simulink model "OPENXWD"  (R2022b)
settings: Solver=VariableStepAuto  StartTime=0.0  StopTime=inf  RelTol=1e-3  EnableMultiTasking=on
PreLoadFcn:
  | run('Parameters\FSE_Parameters.m')
values from neighbouring files (symbols this model uses):
  batt_curr = 1    [srcipt.m]
  batt_voltage = 587    [srcipt.m]
  drive_ratio = 14.25    [srcipt.m]
  g = 9.81    [srcipt.m]
  h = 0.25    [srcipt.m]
  Ku = 1/500*-1    (= -0.002)    [srcipt.m]
  L = 1.53    [srcipt.m]
  lf = L-lr    (= 0.765)    [srcipt.m]
  lr = 0.765    [srcipt.m]
  ls = 1.242    [srcipt.m]
  m = 226    [srcipt.m]
  max_moment = 9.8    [srcipt.m]
  Mz_I = 70    [srcipt.m]
  Mz_p = 700    [srcipt.m]
  P_max = 80000    [srcipt.m]
  rw = 0.217    [srcipt.m]
libraries: CarMaker4SL x44, simulink x1
(part 2 of 3)

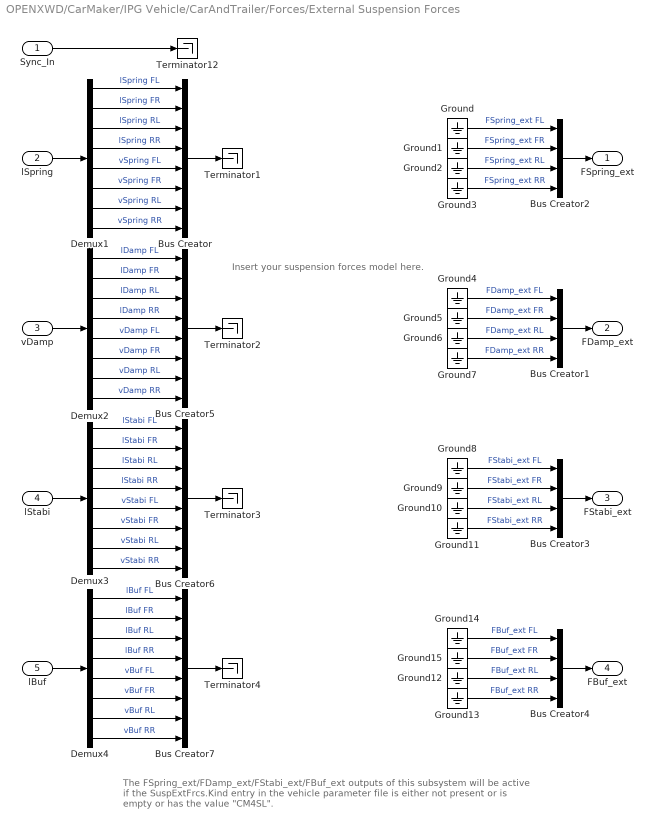
== system OPENXWD/CarMaker/IPG Vehicle/CarAndTrailer/Forces/External Suspension Forces ==
  note: The FSpring_ext/FDamp_ext/FStabi_ext/FBuf_ext outputs of this subsystem will be
      | active if the SuspExtFrcs.Kind entry in the vehicle parameter file
      | is either not present or is empty or has the value "CM4SL".
  note: Insert your suspension forces model here.
  Sync_In : Inport
  lSpring : Inport  Port=2
  vDamp : Inport  Port=3
  lStabi : Inport  Port=4
  lBuf : Inport  Port=5
  Bus Creator{,5..7} (4 alike) : BusCreator  Inputs=8
  Bus Creator{1..4} (4 alike) : BusCreator  Inputs=4
  Demux{1..4} (4 alike) : Demux  Outputs=8
      settings: DisplayOption=none
  Ground{,1..15} (16 alike) : Ground
  Terminator{1..4,12} (5 alike) : Terminator
  FSpring_ext : Outport
  FDamp_ext : Outport  Port=2
  FStabi_ext : Outport  Port=3
  FBuf_ext : Outport  Port=4
  wires:
  Bus Creator7/1 -> Terminator4/1
  Bus Creator6/1 -> Terminator3/1
  Bus Creator5/1 -> Terminator2/1
  Bus Creator/1 -> Terminator1/1
  Demux4/8 -> Bus Creator7/8  "vBuf RR"
  Demux4/7 -> Bus Creator7/7  "vBuf RL"
  Demux4/6 -> Bus Creator7/6  "vBuf FR"
  Demux4/5 -> Bus Creator7/5  "vBuf FL"
  Demux3/8 -> Bus Creator6/8  "vStabi RR"
  Demux3/7 -> Bus Creator6/7  "vStabi RL"
  Demux3/6 -> Bus Creator6/6  "vStabi FR"
  Demux3/5 -> Bus Creator6/5  "vStabi FL"
  Demux2/8 -> Bus Creator5/8  "vDamp RR"
  Demux2/7 -> Bus Creator5/7  "vDamp RL"
  Demux2/6 -> Bus Creator5/6  "vDamp FR"
  Demux2/5 -> Bus Creator5/5  "vDamp FL"
  Demux1/8 -> Bus Creator/8  "vSpring RR"
  Demux1/7 -> Bus Creator/7  "vSpring RL"
  Demux1/6 -> Bus Creator/6  "vSpring FR"
  Demux1/5 -> Bus Creator/5  "vSpring FL"
  Demux2/4 -> Bus Creator5/4  "lDamp RR"
  Demux2/3 -> Bus Creator5/3  "lDamp RL"
  Demux2/2 -> Bus Creator5/2  "lDamp FR"
  Demux2/1 -> Bus Creator5/1  "lDamp FL"
  Demux1/4 -> Bus Creator/4  "lSpring RR"
  Demux1/3 -> Bus Creator/3  "lSpring RL"
  Demux1/2 -> Bus Creator/2  "lSpring FR"
  Demux1/1 -> Bus Creator/1  "lSpring FL"
  Demux3/4 -> Bus Creator6/4  "lStabi RR"
  Demux3/3 -> Bus Creator6/3  "lStabi RL"
  Demux3/2 -> Bus Creator6/2  "lStabi FR"
  Demux3/1 -> Bus Creator6/1  "lStabi FL"
  lStabi/1 -> Demux3/1
  vDamp/1 -> Demux2/1
  lSpring/1 -> Demux1/1
  Demux4/4 -> Bus Creator7/4  "lBuf RR"
  Demux4/3 -> Bus Creator7/3  "lBuf RL"
  Demux4/2 -> Bus Creator7/2  "lBuf FR"
  Demux4/1 -> Bus Creator7/1  "lBuf FL"
  lBuf/1 -> Demux4/1
  Ground14/1 -> Bus Creator4/1  "FBuf_ext FL"
  Ground15/1 -> Bus Creator4/2  "FBuf_ext FR"
  Ground12/1 -> Bus Creator4/3  "FBuf_ext RL"
  Ground13/1 -> Bus Creator4/4  "FBuf_ext RR"
  Bus Creator4/1 -> FBuf_ext/1
  Sync_In/1 -> Terminator12/1
  Bus Creator2/1 -> FSpring_ext/1
  Ground/1 -> Bus Creator2/1  "FSpring_ext FL"
  Ground1/1 -> Bus Creator2/2  "FSpring_ext FR"
  Ground2/1 -> Bus Creator2/3  "FSpring_ext RL"
  Ground3/1 -> Bus Creator2/4  "FSpring_ext RR"
  Ground4/1 -> Bus Creator1/1  "FDamp_ext FL"
  Ground5/1 -> Bus Creator1/2  "FDamp_ext FR"
  Ground6/1 -> Bus Creator1/3  "FDamp_ext RL"
  Ground7/1 -> Bus Creator1/4  "FDamp_ext RR"
  Bus Creator1/1 -> FDamp_ext/1
  Ground8/1 -> Bus Creator3/1  "FStabi_ext FL"
  Ground9/1 -> Bus Creator3/2  "FStabi_ext FR"
  Ground10/1 -> Bus Creator3/3  "FStabi_ext RL"
  Ground11/1 -> Bus Creator3/4  "FStabi_ext RR"
  Bus Creator3/1 -> FStabi_ext/1

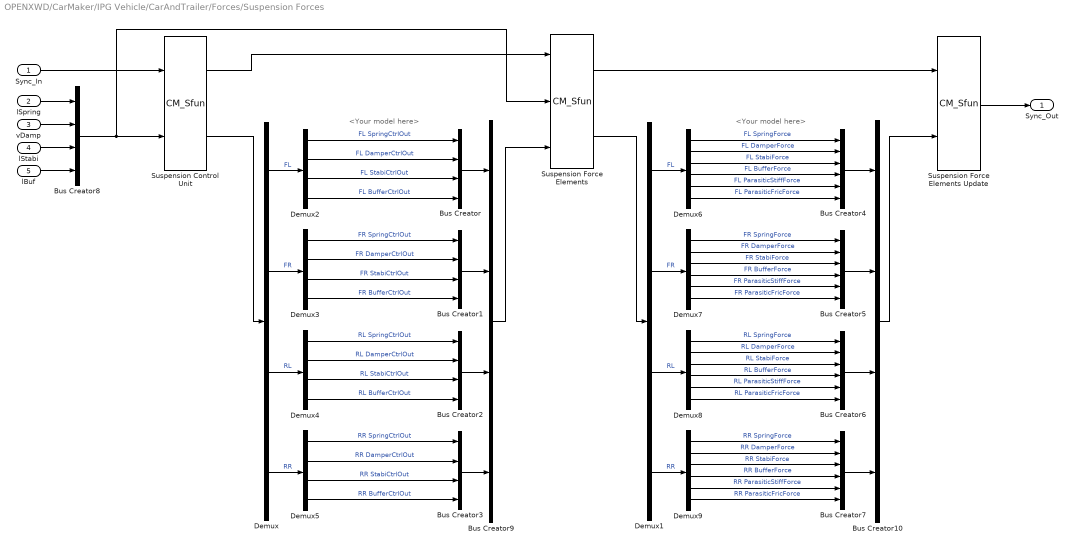
== system OPENXWD/CarMaker/IPG Vehicle/CarAndTrailer/Forces/Suspension Forces ==
  note: <Your model here>
  note: <Your model here>
  Sync_In : Inport
  lSpring : Inport  Port=2
  vDamp : Inport  Port=3
  lStabi : Inport  Port=4
  lBuf : Inport  Port=5
  Bus Creator{,1..3,8..10} (7 alike) : BusCreator  Inputs=4
  Bus Creator{4..7} (4 alike) : BusCreator  Inputs=6
  Demux{,1..5} (6 alike) : Demux
  Demux{6..9} (4 alike) : Demux  Outputs=6
  Suspension Control Unit : S-Function  FunctionName=CM_Sfun  Parameters='ForcesSuspControl'  SFunctionDeploymentMode=off  EnableBusSupport=off
  Suspension Force Elements : S-Function  FunctionName=CM_Sfun  Parameters='ForcesSusp'  SFunctionDeploymentMode=off  EnableBusSupport=off
  Suspension Force Elements Update : S-Function  FunctionName=CM_Sfun  Parameters='ForcesSuspUpd'  SFunctionDeploymentMode=off  EnableBusSupport=off
  Sync_Out : Outport
  wires:
  vDamp/1 -> Bus Creator8/2
  lStabi/1 -> Bus Creator8/3
  lBuf/1 -> Bus Creator8/4
  lSpring/1 -> Bus Creator8/1
  Bus Creator8/1 -> Suspension Control Unit/2, Suspension Force Elements/2
  Sync_In/1 -> Suspension Control Unit/1
  Suspension Control Unit/1 -> Suspension Force Elements/1
  Suspension Force Elements/1 -> Suspension Force Elements Update/1
  Suspension Force Elements Update/1 -> Sync_Out/1
  Bus Creator4/1 -> Bus Creator10/1
  Bus Creator5/1 -> Bus Creator10/2
  Bus Creator6/1 -> Bus Creator10/3
  Bus Creator7/1 -> Bus Creator10/4
  Demux6/1 -> Bus Creator4/1  "FL SpringForce"
  Demux9/1 -> Bus Creator7/1  "RR SpringForce"
  Demux9/2 -> Bus Creator7/2  "RR DamperForce"
  Demux9/3 -> Bus Creator7/3  "RR StabiForce"
  Demux9/4 -> Bus Creator7/4  "RR BufferForce"
  Demux9/5 -> Bus Creator7/5  "RR ParasiticStiffForce"
  Demux9/6 -> Bus Creator7/6  "RR ParasiticFricForce"
  Demux8/1 -> Bus Creator6/1  "RL SpringForce"
  Demux8/2 -> Bus Creator6/2  "RL DamperForce"
  Demux8/4 -> Bus Creator6/4  "RL BufferForce"
  Demux8/5 -> Bus Creator6/5  "RL ParasiticStiffForce"
  Demux8/6 -> Bus Creator6/6  "RL ParasiticFricForce"
  Demux8/3 -> Bus Creator6/3  "RL StabiForce"
  Demux7/1 -> Bus Creator5/1  "FR SpringForce"
  Demux7/2 -> Bus Creator5/2  "FR DamperForce"
  Demux7/3 -> Bus Creator5/3  "FR StabiForce"
  Demux7/4 -> Bus Creator5/4  "FR BufferForce"
  Demux7/5 -> Bus Creator5/5  "FR ParasiticStiffForce"
  Demux7/6 -> Bus Creator5/6  "FR ParasiticFricForce"
  Demux6/2 -> Bus Creator4/2  "FL DamperForce"
  Demux6/3 -> Bus Creator4/3  "FL StabiForce"
  Demux6/4 -> Bus Creator4/4  "FL BufferForce"
  Demux6/5 -> Bus Creator4/5  "FL ParasiticStiffForce"
  Demux6/6 -> Bus Creator4/6  "FL ParasiticFricForce"
  Bus Creator10/1 -> Suspension Force Elements Update/2
  Demux/1 -> Demux2/1  "FL"
  Bus Creator1/1 -> Bus Creator9/2
  Demux/2 -> Demux3/1  "FR"
  Bus Creator2/1 -> Bus Creator9/3
  Demux/3 -> Demux4/1  "RL"
  Bus Creator3/1 -> Bus Creator9/4
  Demux2/1 -> Bus Creator/1  "FL SpringCtrlOut"
  Demux/4 -> Demux5/1  "RR"
  Demux5/1 -> Bus Creator3/1  "RR SpringCtrlOut"
  Demux5/2 -> Bus Creator3/2  "RR DamperCtrlOut"
  Demux5/3 -> Bus Creator3/3  "RR StabiCtrlOut"
  Demux5/4 -> Bus Creator3/4  "RR BufferCtrlOut"
  Demux4/1 -> Bus Creator2/1  "RL SpringCtrlOut"
  Demux4/2 -> Bus Creator2/2  "RL DamperCtrlOut"
  Demux4/4 -> Bus Creator2/4  "RL BufferCtrlOut"
  Demux4/3 -> Bus Creator2/3  "RL StabiCtrlOut"
  Demux3/1 -> Bus Creator1/1  "FR SpringCtrlOut"
  Demux3/2 -> Bus Creator1/2  "FR DamperCtrlOut"
  Demux3/3 -> Bus Creator1/3  "FR StabiCtrlOut"
  Demux3/4 -> Bus Creator1/4  "FR BufferCtrlOut"
  Demux2/2 -> Bus Creator/2  "FL DamperCtrlOut"
  Demux2/3 -> Bus Creator/3  "FL StabiCtrlOut"
  Demux2/4 -> Bus Creator/4  "FL BufferCtrlOut"
  Suspension Control Unit/2 -> Demux/1
  Bus Creator9/1 -> Suspension Force Elements/3
  Bus Creator/1 -> Bus Creator9/1
  Suspension Force Elements/2 -> Demux1/1
  Demux1/1 -> Demux6/1  "FL"
  Demux1/2 -> Demux7/1  "FR"
  Demux1/3 -> Demux8/1  "RL"
  Demux1/4 -> Demux9/1  "RR"

== system OPENXWD/CarMaker/IPG Vehicle/CarAndTrailer/Forces/Tires ==
  note: The TireXX_Out signals will only be used if FileIdent is "CarMaker-Tire-CM4SL" in the tire parameter file!
      | An example parameter file can be found in Data/Tire/DT_CM4SL_UserTire.
  Sync_In : Inport
  TireFL_In : Inport  Port=2
  TireFR_In : Inport  Port=3
  TireRL_In : Inport  Port=4
  TireRR_In : Inport  Port=5
  Bus Creator{1..4} (4 alike) : BusCreator  Inputs=11
  Demux{1..3,8} (4 alike) : Demux  Outputs=7
      settings: DisplayOption=none
  TireFL : Subsystem
  TireFR : Subsystem
  TireRL : Subsystem
  TireRR : Subsystem
  TireFL_Out : Outport
  TireFR_Out : Outport  Port=2
  TireRL_Out : Outport  Port=3
  TireRR_Out : Outport  Port=4
  wires:
  Sync_In/1 -> TireRR/1(Sync_In), TireRL/1(Sync_In), TireFR/1(Sync_In), TireFL/1(Sync_In)
  Bus Creator4/1 -> TireRR_Out/1
  Bus Creator2/1 -> TireRL_Out/1
  Bus Creator1/1 -> TireFR_Out/1
  Demux3/5 -> TireRR/6(Rim_turnv)  "Tire_In Rim_turnv"
  Demux3/4 -> TireRR/5(Rim_rotv)  "Tire_In Rim_rotv"
  Demux3/1 -> TireRR/2(Load)  "Tire_In Load"
  Demux3/7 -> TireRR/8(muRoad)  "Tire_In mu"
  Demux3/6 -> TireRR/7(InclinAngle)  "Tire_In Camber"
  Demux3/2 -> TireRR/3(vxtrans)  "Tire_In vxtrans"
  Demux3/3 -> TireRR/4(vytrans)  "Tire_In vytrans"
  TireRR/11(AlignTrq) -> Bus Creator4/11  "Tire_Out AlignTrq"
  TireRR/10(RollResist) -> Bus Creator4/10  "Tire_Out RollResist"
  TireRR/9(OverturnTrq) -> Bus Creator4/9  "Tire_Out OverturnTrq"
  TireRR/8(LoadFrc) -> Bus Creator4/8  "Tire_Out LoadFrc"
  TireRR/7(SideFrc) -> Bus Creator4/7  "Tire_Out SideFrc"
  TireRR/6(LongFrc) -> Bus Creator4/6  "Tire_Out LongFrc"
  TireRR/5(vBelt) -> Bus Creator4/5  "Tire_Out vBelt"
  TireRR/4(rBelt_eff) -> Bus Creator4/4  "Tire_Out rBelt_eff"
  TireRR/3(TurnSlp) -> Bus Creator4/3  "Tire_Out TurnSlp"
  TireRR/1(Slp) -> Bus Creator4/1  "Tire_Out Slp"
  TireRR/2(Alpha) -> Bus Creator4/2  "Tire_Out Alpha"
  Demux2/5 -> TireRL/6(Rim_turnv)  "Tire_In Rim_turnv"
  Demux2/4 -> TireRL/5(Rim_rotv)  "Tire_In Rim_rotv"
  Demux2/1 -> TireRL/2(Load)  "Tire_In Load"
  Demux2/7 -> TireRL/8(muRoad)  "Tire_In mu"
  Demux2/6 -> TireRL/7(InclinAngle)  "Tire_In Camber"
  Demux2/2 -> TireRL/3(vxtrans)  "Tire_In vxtrans"
  Demux2/3 -> TireRL/4(vytrans)  "Tire_In vytrans"
  TireRL/11(AlignTrq) -> Bus Creator2/11  "Tire_Out AlignTrq"
  TireRL/10(RollResist) -> Bus Creator2/10  "Tire_Out RollResist"
  TireRL/9(OverturnTrq) -> Bus Creator2/9  "Tire_Out OverturnTrq"
  TireRL/8(LoadFrc) -> Bus Creator2/8  "Tire_Out LoadFrc"
  TireRL/7(SideFrc) -> Bus Creator2/7  "Tire_Out SideFrc"
  TireRL/6(LongFrc) -> Bus Creator2/6  "Tire_Out LongFrc"
  TireRL/5(vBelt) -> Bus Creator2/5  "Tire_Out vBelt"
  TireRL/4(rBelt_eff) -> Bus Creator2/4  "Tire_Out rBelt_eff"
  TireRL/3(TurnSlp) -> Bus Creator2/3  "Tire_Out TurnSlp"
  TireRL/1(Slp) -> Bus Creator2/1  "Tire_Out Slp"
  TireRL/2(Alpha) -> Bus Creator2/2  "Tire_Out Alpha"
  Demux1/5 -> TireFR/6(Rim_turnv)  "Tire_In Rim_turnv"
  Demux1/4 -> TireFR/5(Rim_rotv)  "Tire_In Rim_rotv"
  Demux1/1 -> TireFR/2(Load)  "Tire_In Load"
  Demux1/7 -> TireFR/8(muRoad)  "Tire_In mu"
  Demux1/6 -> TireFR/7(InclinAngle)  "Tire_In Camber"
  Demux1/2 -> TireFR/3(vxtrans)  "Tire_In vxtrans"
  Demux1/3 -> TireFR/4(vytrans)  "Tire_In vytrans"
  TireFR/11(AlignTrq) -> Bus Creator1/11  "Tire_Out AlignTrq"
  TireFR/10(RollResist) -> Bus Creator1/10  "Tire_Out RollResist"
  TireFR/9(OverturnTrq) -> Bus Creator1/9  "Tire_Out OverturnTrq"
  TireFR/8(LoadFrc) -> Bus Creator1/8  "Tire_Out LoadFrc"
  TireFR/7(SideFrc) -> Bus Creator1/7  "Tire_Out SideFrc"
  TireFR/6(LongFrc) -> Bus Creator1/6  "Tire_Out LongFrc"
  TireFR/5(vBelt) -> Bus Creator1/5  "Tire_Out vBelt"
  TireFR/4(rBelt_eff) -> Bus Creator1/4  "Tire_Out rBelt_eff"
  TireFR/3(TurnSlp) -> Bus Creator1/3  "Tire_Out TurnSlp"
  TireFR/1(Slp) -> Bus Creator1/1  "Tire_Out Slp"
  TireFR/2(Alpha) -> Bus Creator1/2  "Tire_Out Alpha"
  Demux8/5 -> TireFL/6(Rim_turnv)  "Tire_In Rim_turnv"
  Demux8/4 -> TireFL/5(Rim_rotv)  "Tire_In Rim_rotv"
  TireFL_In/1 -> Demux8/1
  Demux8/1 -> TireFL/2(Load)  "Tire_In Load"
  Demux8/7 -> TireFL/8(muRoad)  "Tire_In mu"
  Demux8/6 -> TireFL/7(InclinAngle)  "Tire_In Camber"
  Demux8/2 -> TireFL/3(vxtrans)  "Tire_In vxtrans"
  Demux8/3 -> TireFL/4(vytrans)  "Tire_In vytrans"
  TireFL/11(AlignTrq) -> Bus Creator3/11  "Tire_Out AlignTrq"
  TireFL/10(RollResist) -> Bus Creator3/10  "Tire_Out RollResist"
  TireFL/9(OverturnTrq) -> Bus Creator3/9  "Tire_Out OverturnTrq"
  TireFL/8(LoadFrc) -> Bus Creator3/8  "Tire_Out LoadFrc"
  TireFL/7(SideFrc) -> Bus Creator3/7  "Tire_Out SideFrc"
  TireFL/6(LongFrc) -> Bus Creator3/6  "Tire_Out LongFrc"
  TireFL/5(vBelt) -> Bus Creator3/5  "Tire_Out vBelt"
  TireFL/4(rBelt_eff) -> Bus Creator3/4  "Tire_Out rBelt_eff"
  TireFL/3(TurnSlp) -> Bus Creator3/3  "Tire_Out TurnSlp"
  TireFL/1(Slp) -> Bus Creator3/1  "Tire_Out Slp"
  TireFL/2(Alpha) -> Bus Creator3/2  "Tire_Out Alpha"
  Bus Creator3/1 -> TireFL_Out/1
  TireFR_In/1 -> Demux1/1
  TireRL_In/1 -> Demux2/1
  TireRR_In/1 -> Demux3/1

== system OPENXWD/CarMaker/IPG Vehicle/CarAndTrailer/Forces/Vehicle Forces ==
  Sync_In : Inport
  Bus Creator1 : BusCreator  Inputs=12
  Bus Creator8 : BusCreator  Inputs=16
  BusCreator1 : BusCreator  Inputs=4
  BusCreator2 : BusCreator  Inputs=9
  DRS_Example : Subsystem
  Demux : Demux  Outputs=16
      settings: DisplayOption=none
  Demux1 : Demux  Outputs=12
      settings: DisplayOption=none
  Demux2 : Demux  Outputs=13
      settings: DisplayOption=none
  Forces : S-Function  FunctionName=CM_Sfun  Parameters='Forces'  SFunctionDeploymentMode=off  EnableBusSupport=off
  Terminator : Terminator
  Sync_Out : Outport
  Car.Virtual : Outport  Port=2
  Car.Aero : Outport  Port=3
  Car.Load : Outport  Port=4
  wires:
  BusCreator1/1 -> Terminator/1  "Aero IF (in)"
  Demux2/13 -> BusCreator2/9  "car Aero Trq_1 z"
  Demux2/12 -> BusCreator2/8  "car Aero Trq_1 y"
  Demux2/11 -> BusCreator2/7  "car Aero Trq_1 x"
  Demux2/7 -> BusCreator2/3  "car Aero PoA_1 z"
  Demux2/6 -> BusCreator2/2  "car Aero PoA_1 y"
  Demux2/5 -> BusCreator2/1  "car Aero PoA_1 x"
  Demux2/4 -> BusCreator1/4  "car Aero tau_1"
  Demux2/3 -> BusCreator1/3  "car Aero ApproachVel_1 z"
  Demux2/2 -> BusCreator1/2  "car Aero ApproachVel_1 y"
  Demux2/1 -> BusCreator1/1  "car Aero ApproachVel_1 x"
  Demux/16 -> Bus Creator8/16  "Car Load_3 tz"
  Demux/15 -> Bus Creator8/15  "Car Load_3 ty"
  Demux/14 -> Bus Creator8/14  "Car Load_3 tx"
  Demux/13 -> Bus Creator8/13  "Car Load_3 mass"
  Demux1/12 -> Bus Creator1/12  "Car Virtual Trq_0 z"
  Demux1/11 -> Bus Creator1/11  "Car Virtual Trq_0 y"
  Demux1/10 -> Bus Creator1/10  "Car Virtual Trq_0 x"
  Demux1/9 -> Bus Creator1/9  "Car Virtual Trq_1 z"
  Demux1/8 -> Bus Creator1/8  "Car Virtual Trq_1 y"
  Demux1/7 -> Bus Creator1/7  "Car Virtual Trq_1 x"
  Demux1/6 -> Bus Creator1/6  "Car Virtual Frc_0 z"
  Demux1/5 -> Bus Creator1/5  "Car Virtual Frc_0 y"
  Demux1/4 -> Bus Creator1/4  "Car Virtual Frc_0 x"
  Sync_In/1 -> Forces/1
  Forces/1 -> Sync_Out/1
  BusCreator2/1 -> Car.Aero/1
  Demux1/1 -> Bus Creator1/1  "Car Virtual Frc_1 x"
  Demux1/2 -> Bus Creator1/2  "Car Virtual Frc_1 y"
  Demux1/3 -> Bus Creator1/3  "Car Virtual Frc_1 z"
  Forces/3 -> Demux2/1
  Forces/2 -> Demux1/1
  Bus Creator1/1 -> Car.Virtual/1
  Bus Creator8/1 -> Car.Load/1
  Demux/1 -> Bus Creator8/1  "Car Load_0 mass"
  Demux/2 -> Bus Creator8/2  "Car Load_0 tx"
  Demux/3 -> Bus Creator8/3  "Car Load_0 ty"
  Demux/4 -> Bus Creator8/4  "Car Load_0 tz"
  Demux/5 -> Bus Creator8/5  "Car Load_1 mass"
  Demux/6 -> Bus Creator8/6  "Car Load_1 tx"
  Demux/7 -> Bus Creator8/7  "Car Load_1 ty"
  Demux/8 -> Bus Creator8/8  "Car Load_1 tz"
  Demux/9 -> Bus Creator8/9  "Car Load_2 mass"
  Demux/10 -> Bus Creator8/10  "Car Load_2 tx"
  Demux/11 -> Bus Creator8/11  "Car Load_2 ty"
  Demux/12 -> Bus Creator8/12  "Car Load_2 tz"
  Forces/4 -> Demux/1
  DRS_Example/1(Car Aero Frc_1x) -> BusCreator2/4
  DRS_Example/2(Car Aero Frc_1y) -> BusCreator2/5
  DRS_Example/3(Car Aero Frc_1z) -> BusCreator2/6

== system OPENXWD/CarMaker/IPG Vehicle/CarAndTrailer/Trailer/CreateBus Car.Hitch.FrcTrq ==
  In1 : Inport
  Bus Creator7 : BusCreator  Inputs=6
  Demux7 : Demux  Outputs=6
      settings: DisplayOption=none
  Out1 : Outport
  wires:
  In1/1 -> Demux7/1
  Bus Creator7/1 -> Out1/1
  Demux7/6 -> Bus Creator7/6  "Car Hitch Trq2Car z"
  Demux7/5 -> Bus Creator7/5  "Car Hitch Trq2Car y"
  Demux7/4 -> Bus Creator7/4  "Car Hitch Trq2Car x"
  Demux7/3 -> Bus Creator7/3  "Car Hitch Frc2Car z"
  Demux7/2 -> Bus Creator7/2  "Car Hitch Frc2Car y"
  Demux7/1 -> Bus Creator7/1  "Car Hitch Frc2Car x"

== system OPENXWD/CarMaker/IPG Vehicle/CarAndTrailer/Trailer/CreateBus Vhcl.Motion ==
  In1 : Inport
  BusCreator : BusCreator  Inputs=15
  Demux : Demux  Outputs=15
      settings: DisplayOption=none
  Out1 : Outport
  wires:
  Demux/15 -> BusCreator/15  "Vhcl YawAcc"
  Demux/14 -> BusCreator/14  "Vhcl YawVel"
  Demux/13 -> BusCreator/13  "Vhcl Yaw"
  Demux/12 -> BusCreator/12  "Vhcl PitchAcc"
  Demux/11 -> BusCreator/11  "Vhcl PitchVel"
  Demux/10 -> BusCreator/10  "Vhcl Pitch"
  Demux/9 -> BusCreator/9  "Vhcl RollAcc"
  Demux/8 -> BusCreator/8  "Vhcl RollVel"
  Demux/7 -> BusCreator/7  "Vhcl Roll"
  Demux/6 -> BusCreator/6  "Vhcl Hitch_Pos z"
  Demux/5 -> BusCreator/5  "Vhcl Hitch_Pos y"
  Demux/4 -> BusCreator/4  "Vhcl Hitch_Pos x"
  Demux/3 -> BusCreator/3  "Vhcl sRoad"
  Demux/2 -> BusCreator/2  "Vhcl Distance"
  Demux/1 -> BusCreator/1  "Vhcl v"
  In1/1 -> Demux/1
  BusCreator/1 -> Out1/1

== system OPENXWD/CarMaker/IPG Vehicle/CarAndTrailer/Trailer/CreateBus Vhcl.PoI ==
  In1 : Inport
  Bus Creator3 : BusCreator  Inputs=18
  Demux3 : Demux  Outputs=18
      settings: DisplayOption=none
  Out1 : Outport
  wires:
  Demux3/18 -> Bus Creator3/18  "Vhcl PoI_GCS Elev"
  Demux3/17 -> Bus Creator3/17  "Vhcl PoI_GCS Lat"
  Demux3/16 -> Bus Creator3/16  "Vhcl PoI_GCS Long"
  Demux3/15 -> Bus Creator3/15  "Vhcl PoI_Acc_1 z"
  Demux3/14 -> Bus Creator3/14  "Vhcl PoI_Acc_1 y"
  Demux3/13 -> Bus Creator3/13  "Vhcl PoI_Acc_1 x"
  Demux3/12 -> Bus Creator3/12  "Vhcl PoI_Vel_1 z"
  Demux3/11 -> Bus Creator3/11  "Vhcl PoI_Vel_1 y"
  Demux3/10 -> Bus Creator3/10  "Vhcl PoI_Vel_1 x"
  Demux3/9 -> Bus Creator3/9  "Vhcl PoI_Acc z"
  Demux3/8 -> Bus Creator3/8  "Vhcl PoI_Acc y"
  Demux3/7 -> Bus Creator3/7  "Vhcl PoI_Acc x"
  Demux3/6 -> Bus Creator3/6  "Vhcl PoI_Vel z"
  Demux3/5 -> Bus Creator3/5  "Vhcl PoI_Vel y"
  Demux3/4 -> Bus Creator3/4  "Vhcl PoI_Vel x"
  Demux3/3 -> Bus Creator3/3  "Vhcl PoI_Pos z"
  Demux3/2 -> Bus Creator3/2  "Vhcl PoI_Pos y"
  In1/1 -> Demux3/1
  Bus Creator3/1 -> Out1/1
  Demux3/1 -> Bus Creator3/1  "Vhcl PoI_Pos x"

== system OPENXWD/CarMaker/IPG Vehicle/CarAndTrailer/Trailer/CreateBus Vhcl.Steering ==
  In1 : Inport
  Bus Creator3 : BusCreator  Inputs=4
  Demux : Demux
      settings: DisplayOption=none
  Out1 : Outport
  wires:
  Bus Creator3/1 -> Out1/1
  Demux/1 -> Bus Creator3/1  "Vhcl Steering Ang"
  Demux/3 -> Bus Creator3/3  "Vhcl Steering AngAcc"
  Demux/2 -> Bus Creator3/2  "Vhcl Steering AngVel"
  Demux/4 -> Bus Creator3/4  "Vhcl Steering Trq"
  In1/1 -> Demux/1

== system OPENXWD/CarMaker/IPG Vehicle/CarAndTrailer/Trailer/CreateBus Vhcl.Wheel.FL ==
  In1 : Inport
  Bus Creator3 : BusCreator  Inputs=14
  Demux3 : Demux  Outputs=14
      settings: DisplayOption=none
  Out1 : Outport
  wires:
  Demux3/14 -> Bus Creator3/14  "Vhcl Wheel FL Trq_WhlBearing"
  Demux3/13 -> Bus Creator3/13  "Vhcl Wheel FL Trq_T2W"
  Demux3/12 -> Bus Creator3/12  "Vhcl Wheel FL SideSlip"
  Demux3/11 -> Bus Creator3/11  "Vhcl Wheel FL LongSlip"
  Demux3/10 -> Bus Creator3/10  "Vhcl Wheel FL vBelt"
  Demux3/9 -> Bus Creator3/9  "Vhcl Wheel FL Fz"
  Demux3/8 -> Bus Creator3/8  "Vhcl Wheel FL Fy"
  Demux3/7 -> Bus Creator3/7  "Vhcl Wheel FL Fx"
  Demux3/6 -> Bus Creator3/6  "Vhcl Wheel FL r_zxy z"
  Demux3/5 -> Bus Creator3/5  "Vhcl Wheel FL r_zxy y"
  Demux3/4 -> Bus Creator3/4  "Vhcl Wheel FL r_zxy x"
  Demux3/3 -> Bus Creator3/3  "Vhcl Wheel FL t z"
  Demux3/2 -> Bus Creator3/2  "Vhcl Wheel FL t y"
  In1/1 -> Demux3/1
  Bus Creator3/1 -> Out1/1
  Demux3/1 -> Bus Creator3/1  "Vhcl Wheel FL t x"

== system OPENXWD/CarMaker/IPG Vehicle/CarAndTrailer/Trailer/CreateBus Vhcl.Wheel.FR ==
  In1 : Inport
  Bus Creator3 : BusCreator  Inputs=14
  Demux3 : Demux  Outputs=14
      settings: DisplayOption=none
  Out1 : Outport
  wires:
  Demux3/14 -> Bus Creator3/14  "Vhcl Wheel FR Trq_WhlBearing"
  Demux3/13 -> Bus Creator3/13  "Vhcl Wheel FR Trq_T2W"
  Demux3/12 -> Bus Creator3/12  "Vhcl Wheel FR SideSlip"
  Demux3/11 -> Bus Creator3/11  "Vhcl Wheel FR LongSlip"
  Demux3/10 -> Bus Creator3/10  "Vhcl Wheel FR vBelt"
  Demux3/9 -> Bus Creator3/9  "Vhcl Wheel FR Fz"
  Demux3/8 -> Bus Creator3/8  "Vhcl Wheel FR Fy"
  Demux3/7 -> Bus Creator3/7  "Vhcl Wheel FR Fx"
  Demux3/6 -> Bus Creator3/6  "Vhcl Wheel FR r_zxy z"
  Demux3/5 -> Bus Creator3/5  "Vhcl Wheel FR r_zxy y"
  Demux3/4 -> Bus Creator3/4  "Vhcl Wheel FR r_zxy x"
  Demux3/3 -> Bus Creator3/3  "Vhcl Wheel FR t z"
  Demux3/2 -> Bus Creator3/2  "Vhcl Wheel FR t y"
  In1/1 -> Demux3/1
  Bus Creator3/1 -> Out1/1
  Demux3/1 -> Bus Creator3/1  "Vhcl Wheel FR t x"

== system OPENXWD/CarMaker/IPG Vehicle/CarAndTrailer/Trailer/CreateBus Vhcl.Wheel.RL ==
  In1 : Inport
  Bus Creator3 : BusCreator  Inputs=14
  Demux3 : Demux  Outputs=14
      settings: DisplayOption=none
  Out1 : Outport
  wires:
  Demux3/14 -> Bus Creator3/14  "Vhcl Wheel RL Trq_WhlBearing"
  Demux3/13 -> Bus Creator3/13  "Vhcl Wheel RL Trq_T2W"
  Demux3/12 -> Bus Creator3/12  "Vhcl Wheel RL SideSlip"
  Demux3/11 -> Bus Creator3/11  "Vhcl Wheel RL LongSlip"
  Demux3/10 -> Bus Creator3/10  "Vhcl Wheel RL vBelt"
  Demux3/9 -> Bus Creator3/9  "Vhcl Wheel RL Fz"
  Demux3/8 -> Bus Creator3/8  "Vhcl Wheel RL Fy"
  Demux3/7 -> Bus Creator3/7  "Vhcl Wheel RL Fx"
  Demux3/6 -> Bus Creator3/6  "Vhcl Wheel RL r_zxy z"
  Demux3/5 -> Bus Creator3/5  "Vhcl Wheel RL r_zxy y"
  Demux3/4 -> Bus Creator3/4  "Vhcl Wheel RL r_zxy x"
  Demux3/3 -> Bus Creator3/3  "Vhcl Wheel RL t z"
  Demux3/2 -> Bus Creator3/2  "Vhcl Wheel RL t y"
  In1/1 -> Demux3/1
  Bus Creator3/1 -> Out1/1
  Demux3/1 -> Bus Creator3/1  "Vhcl Wheel RL t x"

== system OPENXWD/CarMaker/IPG Vehicle/CarAndTrailer/Trailer/CreateBus Vhcl.Wheel.RR ==
  In1 : Inport
  Bus Creator3 : BusCreator  Inputs=14
  Demux3 : Demux  Outputs=14
      settings: DisplayOption=none
  Out1 : Outport
  wires:
  Demux3/14 -> Bus Creator3/14  "Vhcl Wheel RR Trq_WhlBearing"
  Demux3/13 -> Bus Creator3/13  "Vhcl Wheel RR Trq_T2W"
  Demux3/12 -> Bus Creator3/12  "Vhcl Wheel RR SideSlip"
  Demux3/11 -> Bus Creator3/11  "Vhcl Wheel RR LongSlip"
  Demux3/10 -> Bus Creator3/10  "Vhcl Wheel RR vBelt"
  Demux3/9 -> Bus Creator3/9  "Vhcl Wheel RR Fz"
  Demux3/8 -> Bus Creator3/8  "Vhcl Wheel RR Fy"
  Demux3/7 -> Bus Creator3/7  "Vhcl Wheel RR Fx"
  Demux3/6 -> Bus Creator3/6  "Vhcl Wheel RR r_zxy z"
  Demux3/5 -> Bus Creator3/5  "Vhcl Wheel RR r_zxy y"
  Demux3/4 -> Bus Creator3/4  "Vhcl Wheel RR r_zxy x"
  Demux3/3 -> Bus Creator3/3  "Vhcl Wheel RR t z"
  Demux3/2 -> Bus Creator3/2  "Vhcl Wheel RR t y"
  In1/1 -> Demux3/1
  Bus Creator3/1 -> Out1/1
  Demux3/1 -> Bus Creator3/1  "Vhcl Wheel RR t x"

== system OPENXWD/CarMaker/IPG Vehicle/PowerTrain/TorqueVectoring/Reference generator ==
  vx : Inport
  delta : Inport  Port=2
  Constant : Constant
  Divide : Product  Inputs=*/
  Gain1 : Gain  Gain=1/2500
  Product : Product
  Square : Math  Operator=square
  Sum : Sum
  axlebase : Gain  Gain=L
  yaw rate ref : Outport
  wires:
  delta/1 -> Product/1
  Product/1 -> Divide/1
  Constant/1 -> Sum/1
  vx/1 -> Square/1, Product/2  "Vx"
  Square/1 -> Gain1/1
  Gain1/1 -> Sum/2
  Divide/1 -> yaw rate ref/1
  axlebase/1 -> Divide/2
  Sum/1 -> axlebase/1

== system OPENXWD/CarMaker/IPG Vehicle/PowerTrain/TorqueVectoring/Speed estimaor ==
  Input : Inport
  Input1 : Inport  Port=2
  Input2 : Inport  Port=3
  Input3 : Inport  Port=4
  Gain : Gain  Gain=1/4
  Gain1 : Gain  Gain=rw
  Plus : Sum  Inputs=++++
  vx : Outport
  wires:
  Input/1 -> Plus/1
  Input1/1 -> Plus/2
  Input3/1 -> Plus/4
  Input2/1 -> Plus/3
  Plus/1 -> Gain/1
  Gain/1 -> Gain1/1
  Gain1/1 -> vx/1

== system OPENXWD/CarMaker/IPG Vehicle/PowerTrain/TorqueVectoring/Subsystem ==
  Wheel.angle_FL : Inport
  Wheel.angle_FR : Inport  Port=2
  Gain : Gain  Gain=0.5
  Sum : Sum  Inputs=|++
  delta : Outport
  wires:
  Wheel.angle_FL/1 -> Sum/1
  Wheel.angle_FR/1 -> Sum/2
  Sum/1 -> Gain/1
  Gain/1 -> delta/1

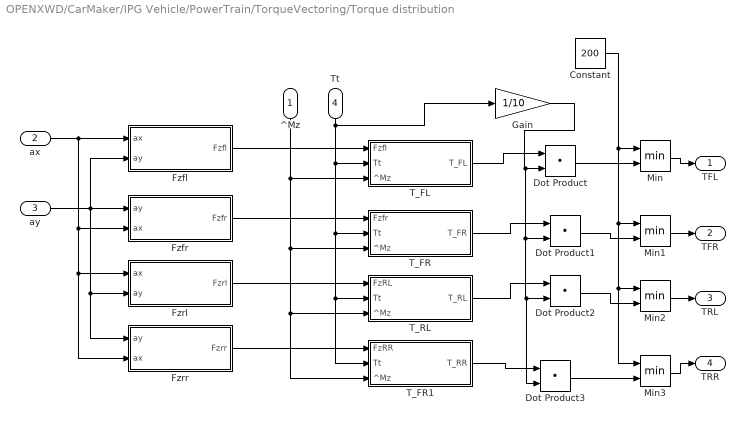
== system OPENXWD/CarMaker/IPG Vehicle/PowerTrain/TorqueVectoring/Torque distribution ==
  ^Mz : Inport
  ax : Inport  Port=2
  ay : Inport  Port=3
  Tt : Inport  Port=4
  Constant : Constant  Value=200
  Dot Product{,1..3} (4 alike) : DotProduct  OutDataTypeStr=Inherit: Inherit via internal rule
  Fzfl : Subsystem
  Fzfr : Subsystem
  Fzrl : Subsystem
  Fzrr : Subsystem
  Gain : Gain  Gain=1/10
  Min{,1..3} (4 alike) : MinMax  Inputs=2
  T_FL : Subsystem
  T_FR : Subsystem
  T_FR1 : Subsystem
  T_RL : Subsystem
  TFL : Outport
  TFR : Outport  Port=2
  TRL : Outport  Port=3
  TRR : Outport  Port=4
  wires:
  ax/1 -> Fzrr/2(ax), Fzrl/1(ax), Fzfr/2(ax), Fzfl/1(ax)
  ay/1 -> Fzfl/2(ay), Fzrr/1(ay), Fzrl/2(ay), Fzfr/1(ay)
  Tt/1 -> Gain/1, T_FR1/2(Tt), T_RL/2(Tt), T_FR/2(Tt), T_FL/2(Tt)
  ^Mz/1 -> T_FR1/3(^Mz), T_RL/3(^Mz), T_FR/3(^Mz), T_FL/3(^Mz)
  Fzfl/1(Fzfl) -> T_FL/1(Fzfl)
  Fzfr/1(Fzfr) -> T_FR/1(Fzfr)
  Fzrl/1(Fzrl) -> T_RL/1(FzRL)
  Fzrr/1(Fzrr) -> T_FR1/1(FzRR)
  T_FL/1(T_FL) -> Dot Product/1
  Gain/1 -> Dot Product3/2, Dot Product2/2, Dot Product1/2, Dot Product/2
  T_FR/1(T_FR) -> Dot Product1/1
  T_RL/1(T_RL) -> Dot Product2/1
  T_FR1/1(T_RR) -> Dot Product3/1
  Constant/1 -> Min3/1, Min2/1, Min1/1, Min/1
  Dot Product/1 -> Min/2
  Min/1 -> TFL/1
  Dot Product3/1 -> Min3/2
  Min3/1 -> TRR/1
  Min2/1 -> TRL/1
  Dot Product2/1 -> Min2/2
  Min1/1 -> TFR/1
  Dot Product1/1 -> Min1/2

== system OPENXWD/CarMaker/IPG Vehicle/PowerTrain/TorqueVectoring/Total Torque Request ==
  acc_pedal : Inport
  brake pedal : Inport  Port=2
  Constant1 : Constant  Value=84
  Product1 : Product
  Sum1 : Sum  Inputs=+-
  Tt : Outport
  wires:
  Sum1/1 -> Product1/2
  Product1/1 -> Tt/1
  acc_pedal/1 -> Sum1/1
  Constant1/1 -> Product1/1
  brake pedal/1 -> Sum1/2

== system OPENXWD/CarMaker/IPG Vehicle/PowerTrain/TorqueVectoring/Upper Controller ==
  yaw rate ref : Inport
  yaw rate : Inport  Port=2
  Gain : Gain  Gain=0.5
  Gain1 : Gain  Gain=0.05
  Integrator : Integrator
  Scope : Scope
  Sum : Sum  Inputs=|-+
  Sum1 : Sum  Inputs=|++
  ^Mz : Outport
  wires:
  yaw rate ref/1 -> Sum/2
  yaw rate/1 -> Sum/1
  Gain1/1 -> Integrator/1
  Integrator/1 -> Sum1/2
  Gain/1 -> Sum1/1
  Sum/1 -> Gain1/1, Gain/1
  Sum1/1 -> Scope/1, ^Mz/1

== system OPENXWD/CarMaker/IPG Vehicle/PowerTrain/TorqueVectoring/Very Important ==
  Constant : Constant  Value=0
  Wind Speed : Outport
  wires:
  Constant/1 -> Wind Speed/1

== system OPENXWD/CarMaker/IPG Vehicle/The Best TorqueVectoring/PowerLimiter/Efficiency ==
  P_mech : Inport
  P_el : Inport  Port=2
  Divide : Product  Inputs=*/
  Output : Outport
  wires:
  P_el/1 -> Divide/2
  Divide/1 -> Output/1
  P_mech/1 -> Divide/1

== system OPENXWD/CarMaker/IPG Vehicle/The Best TorqueVectoring/PowerLimiter/P_mech ==
  Whl_spds : Inport
  Torques : Inport  Port=2
  Demux : Demux
  Demux1 : Demux
  Dot Product{,1..3} (4 alike) : DotProduct  OutDataTypeStr=Inherit: Inherit via internal rule
  Sum : Sum  Inputs=|++++
  P_mech : Outport
  wires:
  Torques/1 -> Demux/1
  Whl_spds/1 -> Demux1/1
  Demux/1 -> Dot Product/1
  Demux1/1 -> Dot Product/2
  Demux1/2 -> Dot Product1/2
  Demux/2 -> Dot Product1/1
  Demux/3 -> Dot Product2/1
  Demux1/3 -> Dot Product2/2
  Demux1/4 -> Dot Product3/2
  Demux/4 -> Dot Product3/1
  Dot Product/1 -> Sum/1
  Dot Product1/1 -> Sum/2
  Dot Product2/1 -> Sum/3
  Dot Product3/1 -> Sum/4
  Sum/1 -> P_mech/1

== system OPENXWD/CarMaker/IPG Vehicle/The Best TorqueVectoring/PowerLimiter/Subsystem ==
  Input : Inport
  Input1 : Inport  Port=2
  Input2 : Inport  Port=3
  Constant : Constant  Value=1000
  Demux : Demux
  Demux1 : Demux
  Divide{,1..3} (4 alike) : Product  Inputs=*/
  Min{,1..3} (4 alike) : MinMax  Inputs=2
  Mux : Mux
  Saturation{,1..3} (4 alike) : Saturate  UpperLimit=inf  LowerLimit=0.5
  Output : Outport
  wires:
  Input/1 -> Demux/1
  Input1/1 -> Demux1/1
  Demux1/4 -> Saturation/1
  Demux1/3 -> Saturation1/1
  Demux1/2 -> Saturation2/1
  Demux1/1 -> Saturation3/1
  Saturation3/1 -> Divide/2
  Saturation/1 -> Divide3/2
  Saturation1/1 -> Divide2/2
  Saturation2/1 -> Divide1/2
  Input2/1 -> Divide3/1, Divide2/1, Divide1/1, Divide/1
  Demux/1 -> Min/1
  Demux/2 -> Min1/1
  Demux/4 -> Min3/1
  Demux/3 -> Min2/1
  Min/1 -> Mux/1
  Min1/1 -> Mux/2
  Min2/1 -> Mux/3
  Min3/1 -> Mux/4
  Mux/1 -> Output/1
  Constant/1 -> Min/2, Min1/2, Min2/2, Min3/2

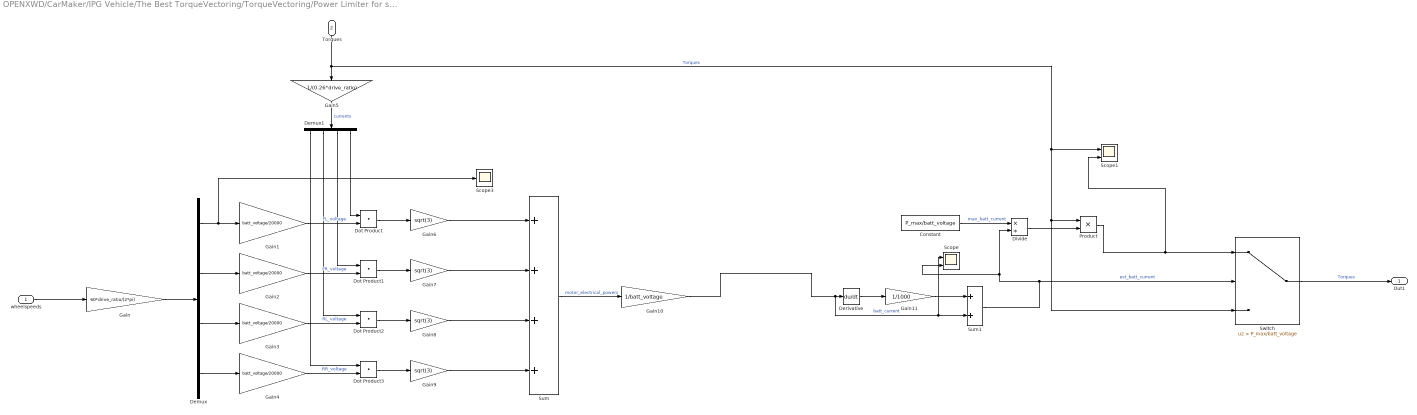
== system OPENXWD/CarMaker/IPG Vehicle/The Best TorqueVectoring/TorqueVectoring/Power Limiter for sim ==
  wheelspeeds : Inport
  Torques : Inport  Port=2  PortDimensions=4
  Constant : Constant  Value=P_max/batt_voltage
  Demux : Demux
  Demux1 : Demux
  Derivative : Derivative
  Divide : Product  Inputs=*/
  Dot Product{,1..3} (4 alike) : DotProduct  OutDataTypeStr=Inherit: Inherit via internal rule
  Gain : Gain  Gain=60*drive_ratio/(2*pi)
  Gain{1..4} (4 alike) : Gain  Gain=batt_voltage/20000
  Gain10 : Gain  Gain=1/batt_voltage
  Gain11 : Gain  Gain=1/1000
  Gain5 : Gain  Gain=1/(0.26*drive_ratio)
  Gain{6..9} (4 alike) : Gain  Gain=sqrt(3)
  Product : Product
  Scope : Scope  NumInputPorts=2
  Scope1 : Scope  NumInputPorts=2
  Scope3 : Scope
  Sum : Sum  Inputs=++++
  Sum1 : Sum
  Switch : Switch  Criteria=u2 > Threshold  Threshold=P_max/batt_voltage  SaturateOnIntegerOverflow=off  InputSameDT=off
  Out1 : Outport
  wires:
  wheelspeeds/1 -> Gain/1
  Gain/1 -> Demux/1
  Demux/1 -> Scope3/1, Gain1/1
  Demux/4 -> Gain4/1
  Demux/3 -> Gain3/1
  Demux/2 -> Gain2/1
  Gain1/1 -> Dot Product/2  "FL_voltage"
  Gain2/1 -> Dot Product1/2  "FR_voltage"
  Gain3/1 -> Dot Product2/2  "RL_voltage"
  Gain4/1 -> Dot Product3/2  "RR_voltage"
  Torques/1 -> Product/1, Switch/3, Scope1/1, Gain5/1  "Torques"
  Gain5/1 -> Demux1/1  "currents"
  Demux1/2 -> Dot Product2/1
  Demux1/1 -> Dot Product3/1
  Dot Product/1 -> Gain6/1
  Dot Product1/1 -> Gain7/1
  Dot Product2/1 -> Gain8/1
  Dot Product3/1 -> Gain9/1
  Gain6/1 -> Sum/1
  Gain7/1 -> Sum/2
  Gain8/1 -> Sum/3
  Gain9/1 -> Sum/4
  Sum/1 -> Gain10/1  "motor_electrical_powers"
  Gain10/1 -> Sum1/2, Scope/1, Derivative/1  "batt_current"
  Derivative/1 -> Gain11/1
  Sum1/1 -> Scope/2, Divide/2, Switch/2  "est_batt_current"
  Constant/1 -> Divide/1  "max_batt_current"
  Divide/1 -> Product/2
  Product/1 -> Scope1/2, Switch/1
  Switch/1 -> Out1/1  "Torques"
  Gain11/1 -> Sum1/1
  Demux1/3 -> Dot Product1/1
  Demux1/4 -> Dot Product/1

== system OPENXWD/CarMaker/IPG Vehicle/The Best TorqueVectoring/TorqueVectoring/Power limiter for car ==
  Torques : Inport
  batt_current : Inport  Port=2
  Constant : Constant  Value=P_max/batt_voltage
  Derivative : Derivative
  Divide : Product  Inputs=*/
  Gain11 : Gain  Gain=1/100
  Product : Product
  Scope : Scope  NumInputPorts=2
  Scope1 : Scope  NumInputPorts=2
  Sum1 : Sum
  Switch : Switch  Criteria=u2 > Threshold  Threshold=P_max/batt_voltage  SaturateOnIntegerOverflow=off  InputSameDT=off
  Torques_lim : Outport
  wires:
  Sum1/1 -> Scope/2, Divide/2, Switch/2  "est_batt_current"
  Gain11/1 -> Sum1/1
  Product/1 -> Scope1/2, Switch/1
  Switch/1 -> Torques_lim/1  "Torques"
  batt_current/1 -> Sum1/2, Scope/1, Derivative/1  "batt_current"
  Derivative/1 -> Gain11/1
  Constant/1 -> Divide/1  "max_batt_current"
  Torques/1 -> Product/1, Switch/3, Scope1/1  "Torques"
  Divide/1 -> Product/2

== system OPENXWD/CarMaker/IPG Vehicle/The Best TorqueVectoring/TorqueVectoring/Reference generator ==
  vx : Inport
  delta : Inport  Port=2
  Constant : Constant
  Desired Understeer Gradient : Gain  Gain=Ku
  Divide : Product  Inputs=*/
  Product : Product
  Saturation : Saturate  UpperLimit=6  LowerLimit=-6
  Saturation1 : Saturate  UpperLimit=inf  LowerLimit=0.3
  Square : Math  Operator=square
  Sum : Sum
  axlebase : Gain  Gain=L
  yaw rate ref : Outport
  wires:
  delta/1 -> Product/1
  Constant/1 -> Sum/1
  vx/1 -> Square/1, Product/2  "Vx"
  Desired Understeer Gradient/1 -> Sum/2
  Sum/1 -> axlebase/1
  Divide/1 -> Saturation/1
  Square/1 -> Desired Understeer Gradient/1
  Product/1 -> Divide/1
  axlebase/1 -> Saturation1/1
  Saturation/1 -> yaw rate ref/1
  Saturation1/1 -> Divide/2

== system OPENXWD/CarMaker/IPG Vehicle/The Best TorqueVectoring/TorqueVectoring/Regenerative braking ==
  note: bezpiecznik temperatury
  note: Negative self alligning torque while braking
  note: We want to maximise driving performance while recuperative braking
  Mz : Inport
  Total Torque : Inport  Port=2
  Constant : Constant  Value=0
  Gain : Gain  Gain=-1
  Manual Switch : ManualSwitch
  Max of Elements : MinMax  Inputs=2
  Subsystem : Subsystem
  Sum : Sum  Inputs=|++
  Switch : Switch  Criteria=u2 > Threshold  SaturateOnIntegerOverflow=off  InputSameDT=off
  Switch1 : Switch  Criteria=u2 > Threshold  SaturateOnIntegerOverflow=off  InputSameDT=off
  Tmax : Subsystem
  Mz_out : Outport
  Tt : Outport  Port=2
  wires:
  Total Torque/1 -> Switch1/2, Switch/1, Switch/2
  Switch/1 -> Tt/1
  Mz/1 -> Gain/1, Switch1/1
  Gain/1 -> Switch1/3
  Switch1/1 -> Mz_out/1
  Subsystem/1(C1) -> Sum/1
  Subsystem/2(C2) -> Sum/2
  Tmax/1(Output) -> Max of Elements/2
  Sum/1 -> Max of Elements/1
  Max of Elements/1 -> Manual Switch/2
  Constant/1 -> Manual Switch/1
  Manual Switch/1 -> Switch/3

== system OPENXWD/CarMaker/IPG Vehicle/The Best TorqueVectoring/TorqueVectoring/Speed estimaor ==
  Input : Inport
  Input1 : Inport  Port=2
  Input2 : Inport  Port=3
  Input3 : Inport  Port=4
  Gain : Gain  Gain=1/4
  Gain1 : Gain  Gain=rw
  Mux : Mux
  Plus : Sum  Inputs=++++
  wheelspeeds : Outport
  vx : Outport  Port=2
  wires:
  Input/1 -> Mux/1, Plus/1
  Input1/1 -> Mux/2, Plus/2
  Input3/1 -> Mux/4, Plus/4
  Input2/1 -> Mux/3, Plus/3
  Plus/1 -> Gain/1
  Gain/1 -> Gain1/1
  Gain1/1 -> vx/1
  Mux/1 -> wheelspeeds/1

== system OPENXWD/CarMaker/IPG Vehicle/The Best TorqueVectoring/TorqueVectoring/Toque distibution NO Tv ==
  Tt : Inport
  Gain : Gain  Gain=1/4
  Mux1 : Mux
  Saturation : Saturate  UpperLimit=inf  LowerLimit=0
  "Const. Torques " : Outport
  wires:
  Tt/1 -> Gain/1
  Gain/1 -> Mux1/2, Mux1/3, Mux1/1, Mux1/4
  Mux1/1 -> Saturation/1
  Saturation/1 -> "Const. Torques "/1

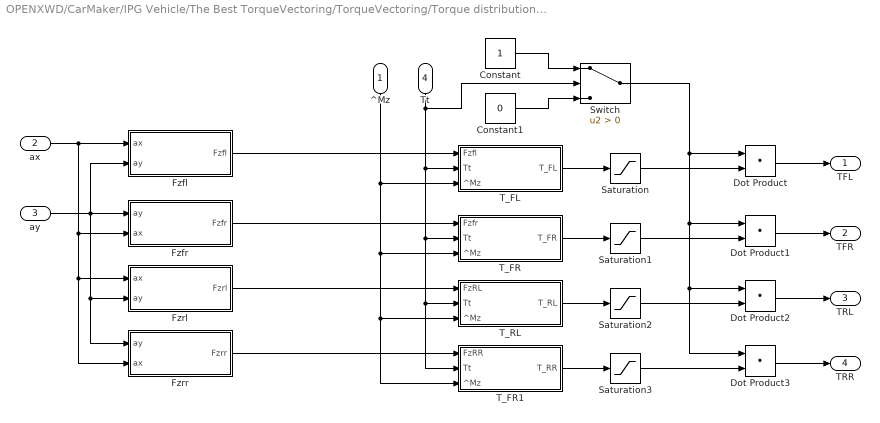
== system OPENXWD/CarMaker/IPG Vehicle/The Best TorqueVectoring/TorqueVectoring/Torque distribution Tv ==
  ^Mz : Inport
  ax : Inport  Port=2
  ay : Inport  Port=3
  Tt : Inport  Port=4
  Constant : Constant
  Constant1 : Constant  Value=0
  Dot Product{,1..3} (4 alike) : DotProduct  OutDataTypeStr=Inherit: Inherit via internal rule
  Fzfl : Subsystem
  Fzfr : Subsystem
  Fzrl : Subsystem
  Fzrr : Subsystem
  Saturation{,1..3} (4 alike) : Saturate  UpperLimit=max_moment*drive_ratio  LowerLimit=-max_moment*drive_ratio
  Switch : Switch  Criteria=u2 > Threshold  SaturateOnIntegerOverflow=off  InputSameDT=off
  T_FL : Subsystem
  T_FR : Subsystem
  T_FR1 : Subsystem
  T_RL : Subsystem
  TFL : Outport
  TFR : Outport  Port=2
  TRL : Outport  Port=3
  TRR : Outport  Port=4
  wires:
  ax/1 -> Fzrr/2(ax), Fzrl/1(ax), Fzfr/2(ax), Fzfl/1(ax)
  ay/1 -> Fzfl/2(ay), Fzrr/1(ay), Fzrl/2(ay), Fzfr/1(ay)
  Tt/1 -> Switch/2, T_FR1/2(Tt), T_RL/2(Tt), T_FR/2(Tt), T_FL/2(Tt)
  ^Mz/1 -> T_FR1/3(^Mz), T_RL/3(^Mz), T_FR/3(^Mz), T_FL/3(^Mz)
  Fzfl/1(Fzfl) -> T_FL/1(Fzfl)
  Fzfr/1(Fzfr) -> T_FR/1(Fzfr)
  Fzrl/1(Fzrl) -> T_RL/1(FzRL)
  Fzrr/1(Fzrr) -> T_FR1/1(FzRR)
  Dot Product/1 -> TFL/1
  Dot Product1/1 -> TFR/1
  Dot Product2/1 -> TRL/1
  Dot Product3/1 -> TRR/1
  T_FL/1(T_FL) -> Saturation/1
  T_FR/1(T_FR) -> Saturation1/1
  T_RL/1(T_RL) -> Saturation2/1
  T_FR1/1(T_RR) -> Saturation3/1
  Constant/1 -> Switch/1
  Constant1/1 -> Switch/3
  Switch/1 -> Dot Product3/1, Dot Product2/1, Dot Product1/1, Dot Product/1
  Saturation/1 -> Dot Product/2
  Saturation1/1 -> Dot Product1/2
  Saturation2/1 -> Dot Product2/2
  Saturation3/1 -> Dot Product3/2

== system OPENXWD/CarMaker/IPG Vehicle/The Best TorqueVectoring/TorqueVectoring/Total Torque Request ==
  acc_pedal : Inport
  Constant : Constant  Value=0
  Constant1 : Constant  Value=4*max_moment*drive_ratio
  Product1 : Product
  Sum1 : Sum  Inputs=+-
  Tt : Outport
  wires:
  Sum1/1 -> Product1/2
  Product1/1 -> Tt/1
  acc_pedal/1 -> Sum1/1
  Constant1/1 -> Product1/1
  Constant/1 -> Sum1/2

== system OPENXWD/CarMaker/IPG Vehicle/The Best TorqueVectoring/TorqueVectoring/Upper Controller ==
  yaw rate ref : Inport
  yaw rate : Inport  Port=2
  Mz Proportional Gain : Inport  Port=3
  Mz Intergative Gain : Inport  Port=4
  Dot Product : DotProduct  OutDataTypeStr=Inherit: Inherit via internal rule
  Dot Product1 : DotProduct  OutDataTypeStr=Inherit: Inherit via internal rule
  Integrator : Integrator
  Sum : Sum  Inputs=|-+
  Sum1 : Sum  Inputs=|++
  ^Mz : Outport
  wires:
  yaw rate ref/1 -> Sum/2
  yaw rate/1 -> Sum/1
  Sum/1 -> Dot Product/2, Dot Product1/1
  Mz Intergative Gain/1 -> Dot Product1/2
  Dot Product/1 -> Sum1/1
  Mz Proportional Gain/1 -> Dot Product/1
  Dot Product1/1 -> Integrator/1
  Integrator/1 -> Sum1/2
  Sum1/1 -> ^Mz/1

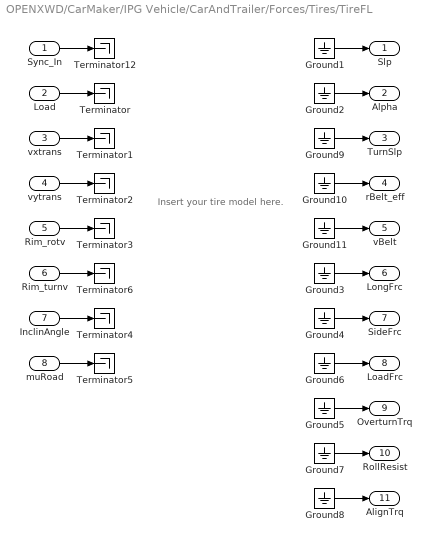
== system OPENXWD/CarMaker/IPG Vehicle/CarAndTrailer/Forces/Tires/TireFL ==
  note: Insert your tire model here.
  Sync_In : Inport
  Load : Inport  Port=2
  vxtrans : Inport  Port=3
  vytrans : Inport  Port=4
  Rim_rotv : Inport  Port=5
  Rim_turnv : Inport  Port=6
  InclinAngle : Inport  Port=7
  muRoad : Inport  Port=8
  Ground{1..11} (11 alike) : Ground
  Terminator{,1..6,12} (8 alike) : Terminator
  Slp : Outport
  Alpha : Outport  Port=2
  TurnSlp : Outport  Port=3
  rBelt_eff : Outport  Port=4
  vBelt : Outport  Port=5
  LongFrc : Outport  Port=6
  SideFrc : Outport  Port=7
  LoadFrc : Outport  Port=8
  OverturnTrq : Outport  Port=9
  RollResist : Outport  Port=10
  AlignTrq : Outport  Port=11
  wires:
  Ground11/1 -> vBelt/1
  Ground10/1 -> rBelt_eff/1
  Ground9/1 -> TurnSlp/1
  Rim_turnv/1 -> Terminator6/1
  Sync_In/1 -> Terminator12/1
  Ground2/1 -> Alpha/1
  Ground3/1 -> LongFrc/1
  Ground4/1 -> SideFrc/1
  Ground5/1 -> OverturnTrq/1
  vxtrans/1 -> Terminator1/1
  vytrans/1 -> Terminator2/1
  Rim_rotv/1 -> Terminator3/1
  InclinAngle/1 -> Terminator4/1
  muRoad/1 -> Terminator5/1
  Load/1 -> Terminator/1
  Ground1/1 -> Slp/1
  Ground6/1 -> LoadFrc/1
  Ground7/1 -> RollResist/1
  Ground8/1 -> AlignTrq/1

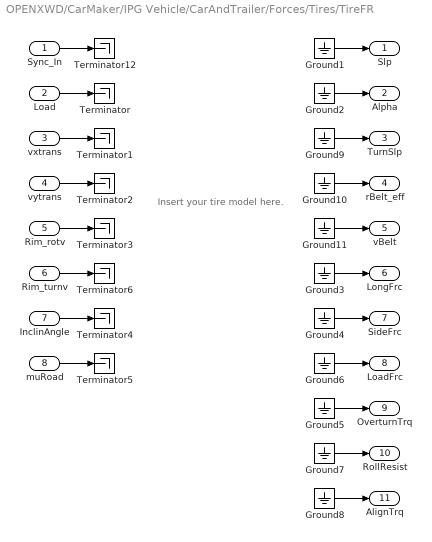
== system OPENXWD/CarMaker/IPG Vehicle/CarAndTrailer/Forces/Tires/TireFR ==
  note: Insert your tire model here.
  Sync_In : Inport
  Load : Inport  Port=2
  vxtrans : Inport  Port=3
  vytrans : Inport  Port=4
  Rim_rotv : Inport  Port=5
  Rim_turnv : Inport  Port=6
  InclinAngle : Inport  Port=7
  muRoad : Inport  Port=8
  Ground{1..11} (11 alike) : Ground
  Terminator{,1..6,12} (8 alike) : Terminator
  Slp : Outport
  Alpha : Outport  Port=2
  TurnSlp : Outport  Port=3
  rBelt_eff : Outport  Port=4
  vBelt : Outport  Port=5
  LongFrc : Outport  Port=6
  SideFrc : Outport  Port=7
  LoadFrc : Outport  Port=8
  OverturnTrq : Outport  Port=9
  RollResist : Outport  Port=10
  AlignTrq : Outport  Port=11
  wires:
  Ground11/1 -> vBelt/1
  Ground10/1 -> rBelt_eff/1
  Ground9/1 -> TurnSlp/1
  Rim_turnv/1 -> Terminator6/1
  Sync_In/1 -> Terminator12/1
  Ground2/1 -> Alpha/1
  Ground3/1 -> LongFrc/1
  Ground4/1 -> SideFrc/1
  Ground5/1 -> OverturnTrq/1
  vxtrans/1 -> Terminator1/1
  vytrans/1 -> Terminator2/1
  Rim_rotv/1 -> Terminator3/1
  InclinAngle/1 -> Terminator4/1
  muRoad/1 -> Terminator5/1
  Load/1 -> Terminator/1
  Ground1/1 -> Slp/1
  Ground6/1 -> LoadFrc/1
  Ground7/1 -> RollResist/1
  Ground8/1 -> AlignTrq/1

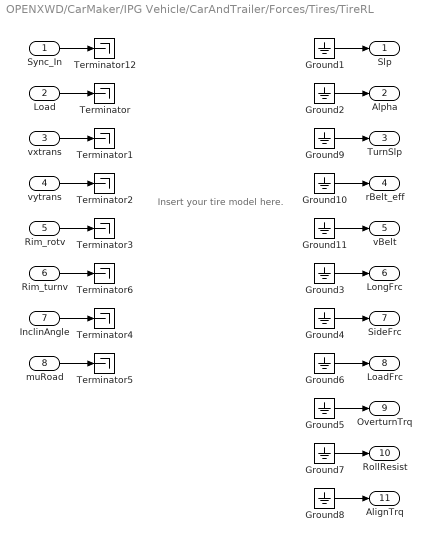
== system OPENXWD/CarMaker/IPG Vehicle/CarAndTrailer/Forces/Tires/TireRL ==
  note: Insert your tire model here.
  Sync_In : Inport
  Load : Inport  Port=2
  vxtrans : Inport  Port=3
  vytrans : Inport  Port=4
  Rim_rotv : Inport  Port=5
  Rim_turnv : Inport  Port=6
  InclinAngle : Inport  Port=7
  muRoad : Inport  Port=8
  Ground{1..11} (11 alike) : Ground
  Terminator{,1..6,12} (8 alike) : Terminator
  Slp : Outport
  Alpha : Outport  Port=2
  TurnSlp : Outport  Port=3
  rBelt_eff : Outport  Port=4
  vBelt : Outport  Port=5
  LongFrc : Outport  Port=6
  SideFrc : Outport  Port=7
  LoadFrc : Outport  Port=8
  OverturnTrq : Outport  Port=9
  RollResist : Outport  Port=10
  AlignTrq : Outport  Port=11
  wires:
  Ground11/1 -> vBelt/1
  Ground10/1 -> rBelt_eff/1
  Ground9/1 -> TurnSlp/1
  Rim_turnv/1 -> Terminator6/1
  Sync_In/1 -> Terminator12/1
  Ground2/1 -> Alpha/1
  Ground3/1 -> LongFrc/1
  Ground4/1 -> SideFrc/1
  Ground5/1 -> OverturnTrq/1
  vxtrans/1 -> Terminator1/1
  vytrans/1 -> Terminator2/1
  Rim_rotv/1 -> Terminator3/1
  InclinAngle/1 -> Terminator4/1
  muRoad/1 -> Terminator5/1
  Load/1 -> Terminator/1
  Ground1/1 -> Slp/1
  Ground6/1 -> LoadFrc/1
  Ground7/1 -> RollResist/1
  Ground8/1 -> AlignTrq/1

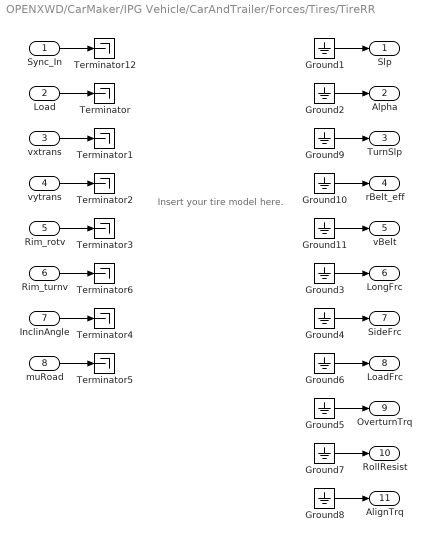
== system OPENXWD/CarMaker/IPG Vehicle/CarAndTrailer/Forces/Tires/TireRR ==
  note: Insert your tire model here.
  Sync_In : Inport
  Load : Inport  Port=2
  vxtrans : Inport  Port=3
  vytrans : Inport  Port=4
  Rim_rotv : Inport  Port=5
  Rim_turnv : Inport  Port=6
  InclinAngle : Inport  Port=7
  muRoad : Inport  Port=8
  Ground{1..11} (11 alike) : Ground
  Terminator{,1..6,12} (8 alike) : Terminator
  Slp : Outport
  Alpha : Outport  Port=2
  TurnSlp : Outport  Port=3
  rBelt_eff : Outport  Port=4
  vBelt : Outport  Port=5
  LongFrc : Outport  Port=6
  SideFrc : Outport  Port=7
  LoadFrc : Outport  Port=8
  OverturnTrq : Outport  Port=9
  RollResist : Outport  Port=10
  AlignTrq : Outport  Port=11
  wires:
  Ground11/1 -> vBelt/1
  Ground10/1 -> rBelt_eff/1
  Ground9/1 -> TurnSlp/1
  Rim_turnv/1 -> Terminator6/1
  Sync_In/1 -> Terminator12/1
  Ground2/1 -> Alpha/1
  Ground3/1 -> LongFrc/1
  Ground4/1 -> SideFrc/1
  Ground5/1 -> OverturnTrq/1
  vxtrans/1 -> Terminator1/1
  vytrans/1 -> Terminator2/1
  Rim_rotv/1 -> Terminator3/1
  InclinAngle/1 -> Terminator4/1
  muRoad/1 -> Terminator5/1
  Load/1 -> Terminator/1
  Ground1/1 -> Slp/1
  Ground6/1 -> LoadFrc/1
  Ground7/1 -> RollResist/1
  Ground8/1 -> AlignTrq/1

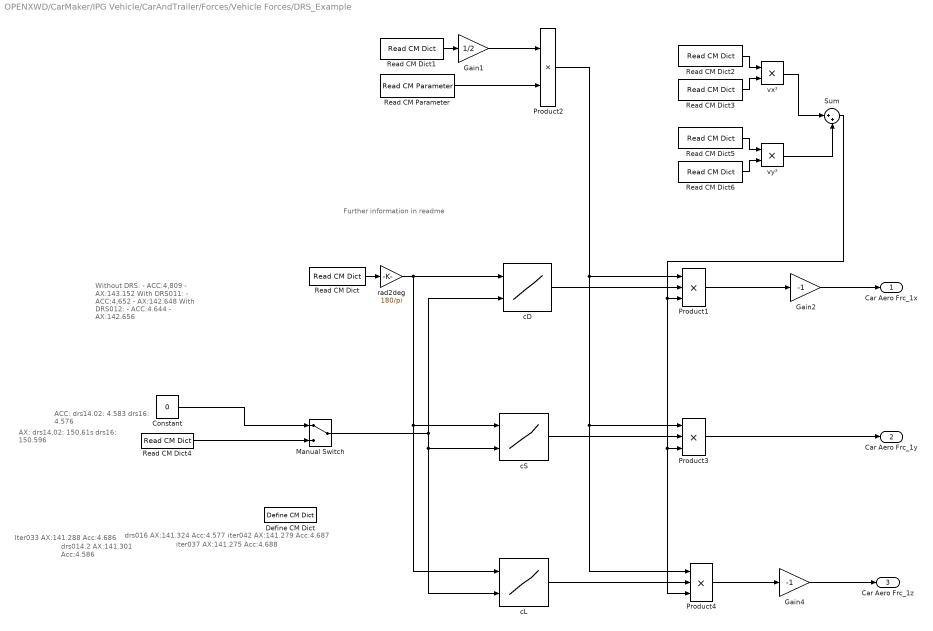
== system OPENXWD/CarMaker/IPG Vehicle/CarAndTrailer/Forces/Vehicle Forces/DRS_Example ==
  note: iter042
      | AX:141.279
      | Acc:4.687
  note: iter037
      | AX:141.275
      | Acc:4.688
  note: drs016
      | AX:141.324
      | Acc:4.577
  note: drs014.2
      | AX:141.301
      | Acc:4.586
  note: Iter033
      | AX:141.288
      | Acc:4.686
  note: ACC:
      | drs14.02:
      | 4.583
      | drs16:
      | 4.576
  note: AX:
      | drs14.02:
      | 150.61s
      | drs16:
      | 150.596
  note: Without DRS:
      | - ACC:4,809
      | - AX:143.152
      | With DRS011:
      | - ACC:4,652
      | - AX:142.648
      | With DRS012:
      | - ACC:4.644
      | - AX:142.656
  note: Further information in readme
  Constant : Constant  Value=0
  Define CM Dict : CarMaker4SL/Define CM Dict  xname=DRS.Switch  xmono=off  xtype=Double4  xdvaplace=IO_In  xnstates=2  xfirststate=0  xinitial=0
  Gain1 : Gain  Gain=1/2
  Gain2 : Gain  Gain=-1
  Gain4 : Gain  Gain=-1
  Manual Switch : ManualSwitch
  Product1 : Product  Inputs=3  RndMeth=Zero
  Product2 : Product  RndMeth=Zero
  Product3 : Product  Inputs=3  RndMeth=Zero
  Product4 : Product  Inputs=3  RndMeth=Zero
  Read CM Dict : CarMaker4SL/Read CM Dict  xname=Car.Aero.tau_1  xsync=off  xstime=Continuous
  Read CM Dict1 : CarMaker4SL/Read CM Dict  xname=Env.AirDensity  xsync=off  xstime=Continuous
  Read CM Dict2 : CarMaker4SL/Read CM Dict  xname=Car.Aero.vres_1.x  xsync=off  xstime=Continuous
  Read CM Dict3 : CarMaker4SL/Read CM Dict  xname=Car.Aero.vres_1.x  xsync=off  xstime=Continuous
  Read CM Dict4 : CarMaker4SL/Read CM Dict  xname=DRS.Switch  xsync=off  xstime=Continuous
  Read CM Dict5 : CarMaker4SL/Read CM Dict  xname=Car.Aero.vres_1.y  xsync=off  xstime=Continuous
  Read CM Dict6 : CarMaker4SL/Read CM Dict  xname=Car.Aero.vres_1.y  xsync=off  xstime=Continuous
  Read CM Parameter : CarMaker4SL/Read CM Parameter  xfile=Vehicle  xkey=Aero.Ax  xnout=1  xdefaults=0  xmuxed=on  xstime=Continuous
      settings: SourceProductName=CarMaker4SL
  Sum : Sum  Inputs=|++
  cD : Lookup_n-D  BreakpointsForDimension1=AeroFD(2:end, 1)  BreakpointsForDimension2=AeroFD(1, 2:end)  Table=AeroFD(2:end, 2:end)  RndMeth=Simplest
      settings: InputPortMap=u0,u1
  cL : Lookup_n-D  BreakpointsForDimension1=AeroFL(2:end, 1)  BreakpointsForDimension2=AeroFL(1, 2:end)  Table=AeroFL(2:end, 2:end)  RndMeth=Simplest
      settings: InputPortMap=u0,u1
  cS : Lookup_n-D  BreakpointsForDimension1=AeroFS(2:end, 1)  BreakpointsForDimension2=AeroFS(1, 2:end)  Table=AeroFS(2:end, 2:end)  RndMeth=Simplest
      settings: InputPortMap=u0,u1
  rad2deg : Gain  Gain=180/pi
  vx² : Product  RndMeth=Zero
  vy² : Product  RndMeth=Zero
  Car Aero Frc_1x : Outport  VectorParamsAs1DForOutWhenUnconnected=off
  Car Aero Frc_1y : Outport  Port=2  VectorParamsAs1DForOutWhenUnconnected=off
  Car Aero Frc_1z : Outport  Port=3  VectorParamsAs1DForOutWhenUnconnected=off
  wires:
  Read CM Dict/1 -> rad2deg/1
  Read CM Dict1/1 -> Gain1/1
  Read CM Dict2/1 -> vx²/1
  Read CM Dict3/1 -> vx²/2
  Gain1/1 -> Product2/1
  Gain2/1 -> Car Aero Frc_1x/1
  Gain4/1 -> Car Aero Frc_1z/1
  Product2/1 -> Product1/1, Product3/1, Product4/1
  Product1/1 -> Gain2/1
  Read CM Parameter/1 -> Product2/2
  rad2deg/1 -> cD/1, cS/1, cL/1
  Manual Switch/1 -> cD/2, cL/2, cS/2
  Product3/1 -> Car Aero Frc_1y/1
  Product4/1 -> Gain4/1
  Read CM Dict5/1 -> vy²/1
  Read CM Dict6/1 -> vy²/2
  cD/1 -> Product1/2
  cS/1 -> Product3/2
  cL/1 -> Product4/2
  vx²/1 -> Sum/1
  vy²/1 -> Sum/2
  Sum/1 -> Product1/3, Product3/3, Product4/3
  Constant/1 -> Manual Switch/1
  Read CM Dict4/1 -> Manual Switch/2

== system OPENXWD/CarMaker/IPG Vehicle/PowerTrain/TorqueVectoring/Torque distribution/Fzfl ==
  ax : Inport
  ay : Inport  Port=2
  Constant : Constant  Value=g*lr
  Gain : Gain  Gain=m/(2*L)
  Gain1 : Gain  Gain=h
  Gain2 : Gain  Gain=(h*lr)/(ls)
  Sum : Sum  Inputs=+--
  Fzfl : Outport
  wires:
  Sum/1 -> Gain/1
  Constant/1 -> Sum/1
  Gain1/1 -> Sum/2
  ax/1 -> Gain1/1
  ay/1 -> Gain2/1
  Gain2/1 -> Sum/3
  Gain/1 -> Fzfl/1

== system OPENXWD/CarMaker/IPG Vehicle/PowerTrain/TorqueVectoring/Torque distribution/Fzfr ==
  ay : Inport
  ax : Inport  Port=2
  Constant : Constant  Value=g*lr
  Gain : Gain  Gain=m/(2*L)
  Gain1 : Gain  Gain=h
  Gain2 : Gain  Gain=(h*lr)/(ls)
  Sum : Sum  Inputs=+-+
  Fzfr : Outport
  wires:
  Sum/1 -> Gain/1
  Constant/1 -> Sum/1
  Gain1/1 -> Sum/2
  ax/1 -> Gain1/1
  ay/1 -> Gain2/1
  Gain2/1 -> Sum/3
  Gain/1 -> Fzfr/1

== system OPENXWD/CarMaker/IPG Vehicle/PowerTrain/TorqueVectoring/Torque distribution/Fzrl ==
  ax : Inport
  ay : Inport  Port=2
  Constant : Constant  Value=g*lf
  Gain : Gain  Gain=m/(2*L)
  Gain1 : Gain  Gain=h
  Gain2 : Gain  Gain=(h*lf)/(ls)
  Sum : Sum  Inputs=++-
  Fzrl : Outport
  wires:
  Gain/1 -> Fzrl/1
  Gain2/1 -> Sum/3
  ay/1 -> Gain2/1
  Sum/1 -> Gain/1
  Constant/1 -> Sum/1
  ax/1 -> Gain1/1
  Gain1/1 -> Sum/2

== system OPENXWD/CarMaker/IPG Vehicle/PowerTrain/TorqueVectoring/Torque distribution/Fzrr ==
  ay : Inport
  ax : Inport  Port=2
  Constant : Constant  Value=g*lf
  Gain : Gain  Gain=m/(2*L)
  Gain1 : Gain  Gain=h
  Gain2 : Gain  Gain=(h*lf)/(ls)
  Sum : Sum  Inputs=+++
  Fzrr : Outport
  wires:
  Gain/1 -> Fzrr/1
  Gain2/1 -> Sum/3
  ay/1 -> Gain2/1
  Sum/1 -> Gain/1
  Constant/1 -> Sum/1
  ax/1 -> Gain1/1
  Gain1/1 -> Sum/2

== system OPENXWD/CarMaker/IPG Vehicle/PowerTrain/TorqueVectoring/Torque distribution/T_FL ==
  Fzfl : Inport
  Tt : Inport  Port=2
  ^Mz : Inport  Port=3
  Gain : Gain  Gain=rw/ls
  Gain1 : Gain  Gain=1/(m*g)
  Product : Product
  Sum : Sum  Inputs=+-
  T_FL : Outport
  wires:
  Gain/1 -> Sum/2
  Tt/1 -> Sum/1
  ^Mz/1 -> Gain/1
  Fzfl/1 -> Gain1/1
  Gain1/1 -> Product/1
  Product/1 -> T_FL/1
  Sum/1 -> Product/2

== system OPENXWD/CarMaker/IPG Vehicle/PowerTrain/TorqueVectoring/Torque distribution/T_FR ==
  Fzfr : Inport
  Tt : Inport  Port=2
  ^Mz : Inport  Port=3
  Gain : Gain  Gain=rw/ls
  Gain1 : Gain  Gain=1/(m*g)
  Product : Product
  Sum : Sum
  T_FR : Outport
  wires:
  Gain/1 -> Sum/2
  Tt/1 -> Sum/1
  ^Mz/1 -> Gain/1
  Fzfr/1 -> Gain1/1
  Gain1/1 -> Product/1
  Product/1 -> T_FR/1
  Sum/1 -> Product/2

== system OPENXWD/CarMaker/IPG Vehicle/PowerTrain/TorqueVectoring/Torque distribution/T_FR1 ==
  FzRR : Inport
  Tt : Inport  Port=2
  ^Mz : Inport  Port=3
  Gain : Gain  Gain=rw/ls
  Gain1 : Gain  Gain=1/(m*g)
  Product : Product
  Sum : Sum
  T_RR : Outport
  wires:
  Gain/1 -> Sum/2
  Tt/1 -> Sum/1
  ^Mz/1 -> Gain/1
  FzRR/1 -> Gain1/1
  Gain1/1 -> Product/1
  Product/1 -> T_RR/1
  Sum/1 -> Product/2

== system OPENXWD/CarMaker/IPG Vehicle/PowerTrain/TorqueVectoring/Torque distribution/T_RL ==
  FzRL : Inport
  Tt : Inport  Port=2
  ^Mz : Inport  Port=3
  Gain : Gain  Gain=rw/ls
  Gain1 : Gain  Gain=1/(m*g)
  Product : Product
  Sum : Sum  Inputs=+-
  T_RL : Outport
  wires:
  Gain/1 -> Sum/2
  Tt/1 -> Sum/1
  ^Mz/1 -> Gain/1
  FzRL/1 -> Gain1/1
  Gain1/1 -> Product/1
  Product/1 -> T_RL/1
  Sum/1 -> Product/2

== system OPENXWD/CarMaker/IPG Vehicle/The Best TorqueVectoring/TorqueVectoring/Regenerative braking/Subsystem ==
  Gain : Gain  Gain=1/drive_ratio
  Gain1 : Gain  Gain=1/drive_ratio
  Ta : Gain  Gain=rw
  Tr : Gain  Gain=rw
  X1 : Gain  Gain=1.3
  X2 : Gain  Gain=1.3
  Z1 : Constant  Value=(m*g*lf)/L
  Z2 : Constant  Value=(m*g*lr)/L
  C1 : Outport
  C2 : Outport  Port=2
  wires:
  Z1/1 -> X1/1
  Z2/1 -> X2/1
  X1/1 -> Ta/1
  X2/1 -> Tr/1
  Ta/1 -> Gain/1
  Tr/1 -> Gain1/1
  Gain/1 -> C1/1
  Gain1/1 -> C2/1
